simulink library "nested_mask"  (R2017b)
settings: Solver=VariableStepAuto  StartTime=0.0  StopTime=10.0  RelTol=1e-3
libraries: nested_mask x2
settings Model: Creator=cyarp  LastModifiedBy=cyarp

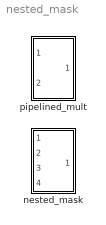
== system nested_mask ==
  nested_mask : Subsystem  mask{mul=0, ad=0}
      mask prompts: mul "Mult Delay"; ad "Add Delay"
  pipelined_mult : Subsystem  mask{mult_delay=0}
      mask prompts: mult_delay "Multiplication Delay"

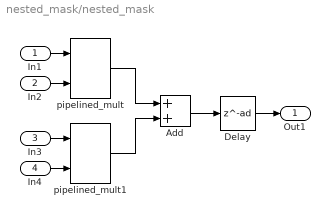
== system nested_mask/nested_mask ==
  In1 : Inport
  In2 : Inport  Port=2
  In3 : Inport  Port=3
  In4 : Inport  Port=4
  Add : Sum
  Delay : Delay  DelayLength=ad
  pipelined_mult : nested_mask/pipelined_mult  mult_delay=mul+1
  pipelined_mult1 : nested_mask/pipelined_mult  mult_delay=mul+1
  Out1 : Outport
  wires:
  In4/1 -> pipelined_mult1/2
  pipelined_mult/1 -> Add/1
  In2/1 -> pipelined_mult/2
  In1/1 -> pipelined_mult/1
  Delay/1 -> Out1/1
  Add/1 -> Delay/1
  In3/1 -> pipelined_mult1/1
  pipelined_mult1/1 -> Add/2

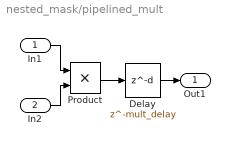
== system nested_mask/pipelined_mult ==
  In1 : Inport
  In2 : Inport  Port=2
  Delay : Delay  DelayLength=mult_delay  InitialCondition=0
  Product : Product
  Out1 : Outport
  wires:
  Product/1 -> Delay/1
  In2/1 -> Product/2
  Delay/1 -> Out1/1
  In1/1 -> Product/1
